simulink model "Nonlinear_equations"  (R2022b)
settings: Solver=ode4  StartTime=0.0  StopTime=10.0  FixedStep=0.001  RelTol=1e-3
undefined symbols (not defined in the file): c, f, g, J, Kb, Km, Ku, L, M, Nr, r, Ra
settings Model: Creator=shuan  LastModifiedBy=X1
settings SolverCC: AlgebraicLoopSolver=TrustRegion
settings DebuggingCC: SFMachineParentedDataDiag=warning

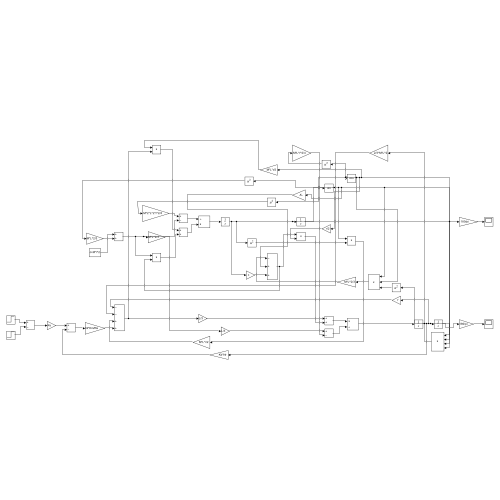
[thumbnail: Simulink's stored preview of the top-level diagram]
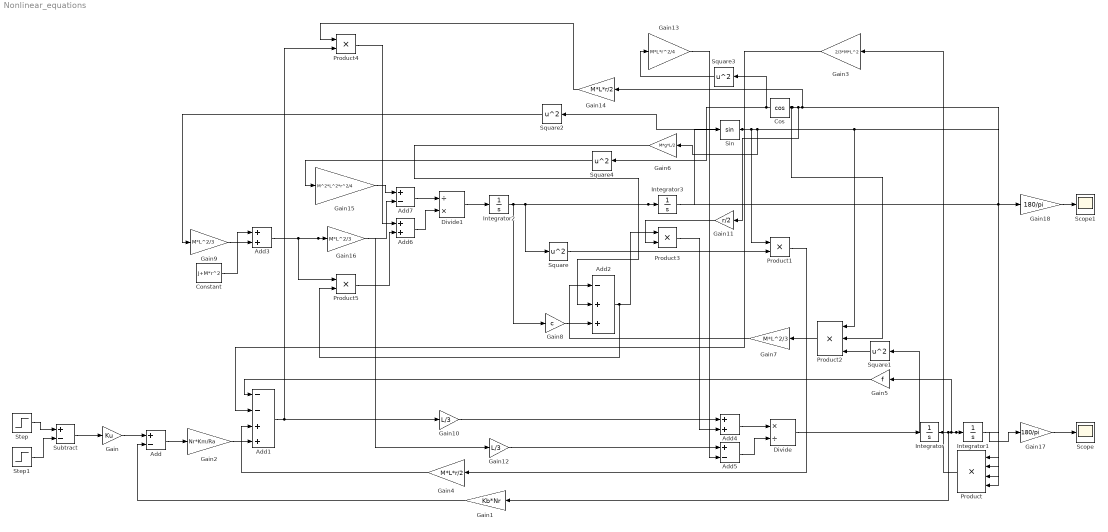
== system Nonlinear_equations ==
  Add : Sum  Inputs=+-
  Add1 : Sum  Inputs=--++
  Add2 : Sum  Inputs=-++
  Add3 : Sum
  Add4 : Sum
  Add5 : Sum  Inputs=+-
  Add6 : Sum
  Add7 : Sum  Inputs=+-
  Constant : Constant  Value=J+M*r^2
  Cos : Trigonometry  Operator=cos
  Divide : Product  Inputs=*/
  Divide1 : Product  Inputs=/*
  Gain : Gain  Gain=Ku
  Gain1 : Gain  Gain=Kb*Nr
  Gain10 : Gain  Gain=L/3
  Gain11 : Gain  Gain=r/2
  Gain12 : Gain  Gain=L/3
  Gain13 : Gain  Gain=M*L*r^2/4
  Gain14 : Gain  Gain=M*L*r/2
  Gain15 : Gain  Gain=M^2*L^2*r^2/4
  Gain16 : Gain  Gain=M*L^2/3
  Gain17 : Gain  Gain=180/pi
  Gain18 : Gain  Gain=180/pi
  Gain2 : Gain  Gain=Nr*Km/Ra
  Gain3 : Gain  Gain=2/3*M*L^2
  Gain4 : Gain  Gain=M*L*r/2
  Gain5 : Gain  Gain=f
  Gain6 : Gain  Gain=M*g*L/2
  Gain7 : Gain  Gain=M*L^2/3
  Gain8 : Gain  Gain=c
  Gain9 : Gain  Gain=M*L^2/3
  Integrator{,1..3} (4 alike) : Integrator
  Product : Product  Inputs=4
  Product{1,3..5} (4 alike) : Product
  Product2 : Product  Inputs=3
  Scope : Scope
  Scope1 : Scope
  Sin : Trigonometry
  Square{,1..4} (5 alike) : Math  Operator=square
  Step : Step  Time=0  SampleTime=0
  Step1 : Step  Time=0.1  SampleTime=0
  Subtract : Sum  Inputs=+-
  wires:
  Integrator2/1 -> Integrator3/1, Product/3, Square/1, Gain8/1
  Subtract/1 -> Gain/1
  Integrator3/1 -> Sin/1
  Gain/1 -> Add/1
  Add/1 -> Gain2/1
  Square1/1 -> Product2/3
  Gain6/1 -> Add2/2
  Gain9/1 -> Add3/2
  Gain18/1 -> Scope1/1
  Sin/1 -> Product/1, Product2/1, Gain6/1, Product1/1, Square2/1
  Constant/1 -> Add3/1
  Add1/1 -> Gain10/1, Product4/2
  Gain17/1 -> Scope/1
  Gain1/1 -> Add/2
  Gain2/1 -> Add1/4
  Add4/1 -> Divide/1
  Product3/1 -> Add4/2
  Add3/1 -> Gain16/1, Gain12/1, Product5/1
  Add5/1 -> Divide/2
  Square2/1 -> Gain9/1
  Product5/1 -> Add6/2
  Product4/1 -> Add6/1
  Product2/1 -> Gain7/1
  Gain10/1 -> Add4/1
  Add6/1 -> Divide1/2
  Gain15/1 -> Add7/1
  Integrator/1 -> Product/4, Integrator1/1, Gain5/1, Gain1/1, Square1/1
  Gain16/1 -> Add7/2
  Divide1/1 -> Integrator2/1
  Add7/1 -> Divide1/1
  Product/1 -> Gain3/1
  Gain3/1 -> Add1/2
  Product1/1 -> Gain4/1
  Gain4/1 -> Add1/3
  Divide/1 -> Integrator/1
  Square3/1 -> Gain13/1
  Gain13/1 -> Add5/2
  Square/1 -> Product1/2
  Gain12/1 -> Add5/1
  Gain7/1 -> Add2/1
  Gain8/1 -> Add2/3
  Gain11/1 -> Product3/2
  Square4/1 -> Gain15/1
  Gain14/1 -> Product4/1
  Add2/1 -> Product5/2, Product3/1
  Cos/1 -> Gain14/1, Product/2, Gain18/1, Gain11/1, Square4/1, Square3/1, Product2/2
  Gain5/1 -> Add1/1
  Integrator1/1 -> Gain17/1
  Step/1 -> Subtract/1
  Step1/1 -> Subtract/2
